simulink model "ask"  (R2018a)
settings: Solver=VariableStepAuto  StartTime=0.0  StopTime=10  RelTol=1e-3
libraries: commchan3 x1, simulink x1, dspfdesign x1, commseqgen3 x1
settings Model: Creator=Владимир  LastModifiedBy=Владимир

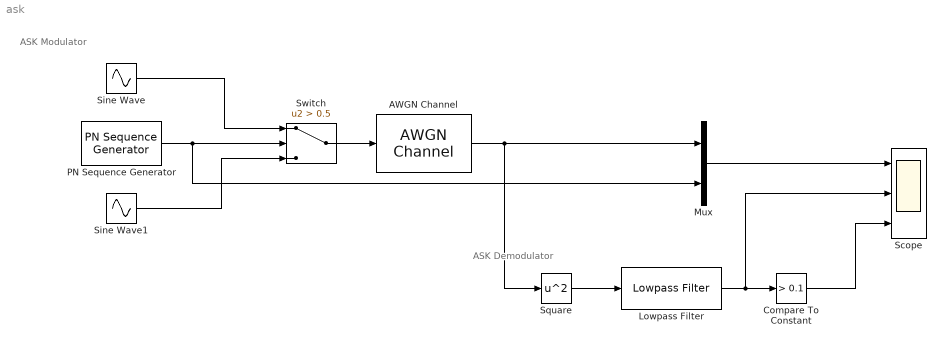
== system ask ==
  note: ASK Demodulator
  note: ASK Modulator
  AWGN Channel : commchan3/AWGN Channel  InputProcessing=Columns as channels (frame based)  seed=67  noiseMode="Signal to noise ratio  (SNR)"  EbNodB=40  EsNodB=10  SNRdB=30  bitsPerSym=1  Ps=1  Tsym=1  variance=1
  Compare To Constant : simulink/Logic and Bit Operations/Compare To Constant  relop=>  const=0.1  OutDataTypeStr=boolean
  Lowpass Filter : dspfdesign/Lowpass Filter  FilterType=FIR  DesignForMinimumOrder=on  FilterOrder=50  PassbandFrequency=2  StopbandFrequency=4  PassbandRipple=1  StopbandAttenuation=60  InheritSampleRate=on  SampleRate=1000  SimulateUsing=Interpreted execution  roundingMode=Floor  coeffsDataTypeStr=fixdt(1,16)
  Mux : Mux  Inputs=2
  PN Sequence Generator : commseqgen3/PN Sequence Generator  poly='z^6 + z + 1'  ini_sta=[0 0 0 1 0 1]  outBitMaskSource=Dialog parameter  shift=0  outVarSiz=off  maxOutSizeMode=Dialog parameter  maxOutSize=[10 1]  Ts=1  sampPerFrame=1  reset=off  bitPackedOutputs=off  outDataType=double  numPackedBits=8  bitPackDataSigned=off  bitPackedOutDType=double
      settings: SourceProductName=Communications System Toolbox
  Scope : Scope  NumInputPorts=3
  Sine Wave : Sin  Frequency=2*pi*10  SampleTime=0.001
  Sine Wave1 : Sin  Amplitude=0.1  Frequency=2*pi*10  SampleTime=0.001
  Square : Math  Operator=square  SaturateOnIntegerOverflow=on
  Switch : Switch  Criteria=u2 > Threshold  Threshold=0.5
  wires:
  PN Sequence Generator/1 -> Mux/2, Switch/2
  Switch/1 -> AWGN Channel/1
  Mux/1 -> Scope/1
  Sine Wave/1 -> Switch/1
  Sine Wave1/1 -> Switch/3
  Square/1 -> Lowpass Filter/1
  AWGN Channel/1 -> Square/1, Mux/1
  Compare To Constant/1 -> Scope/3
  Lowpass Filter/1 -> Compare To Constant/1, Scope/2
